simulink model "Hybrid_powertrain"  (R2021b)
settings: Solver=VariableStepAuto  StartTime=0.0  StopTime=1801  RelTol=1e-3
undefined symbols (not defined in the file): A, bvolt, C_d, discharge_mah, eff_bat, eff_dt, Eff_map, eff_map, f_rr, g, i, id, m, magnitude, Max_Torque, mu, P_aux, PM_max, r_d, rho, Ri_bat, soc_start, spd, Speed, TM_max, Torque, torque, v_reg_lim, wM_base
libraries: simulink x1, slpidlib x1
settings Model: Creator=Admin  LastModifiedBy=Admin

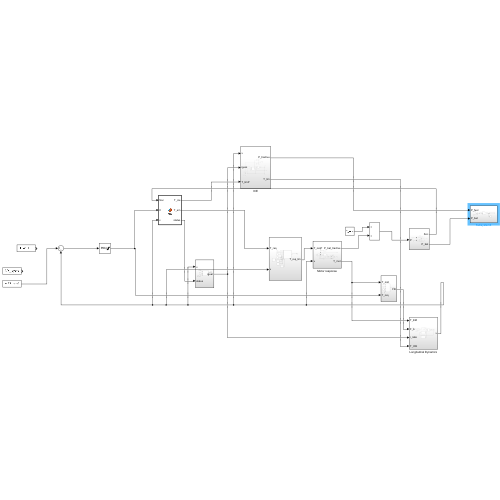
[thumbnail: Simulink's stored preview of the top-level diagram]
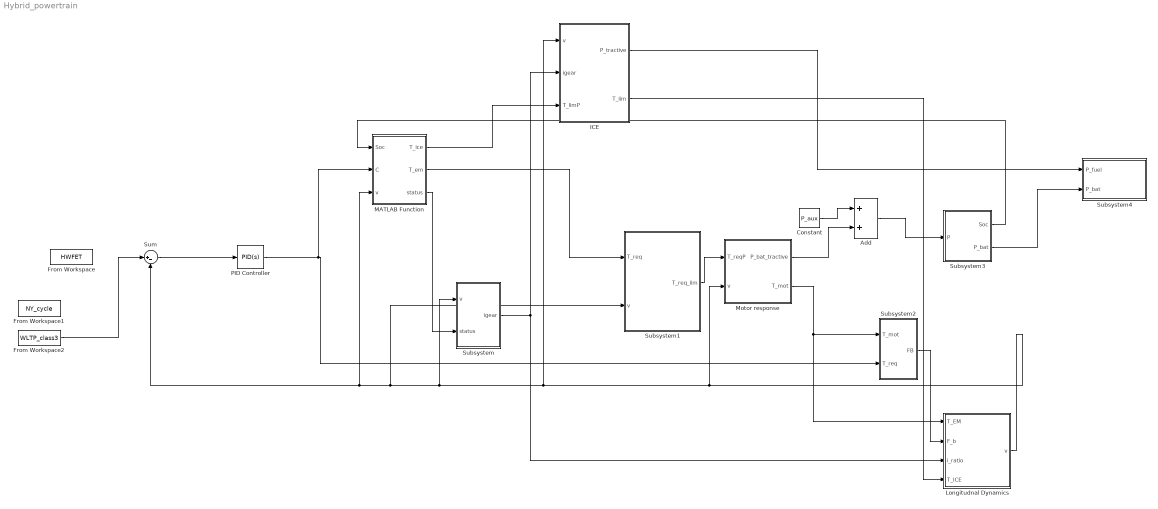
== system Hybrid_powertrain ==
  Add : Sum
  Constant : Constant  Value=P_aux
  From Workspace : FromWorkspace  VariableName=HWFET
  From Workspace1 : FromWorkspace  VariableName=NY_cycle
  From Workspace2 : FromWorkspace  VariableName=WLTP_class3
  ICE : Subsystem
  Longitudnal Dynamics : Subsystem
  MATLAB Function : MATLAB Function  TreatAsAtomicUnit=on
  Motor response : Subsystem
  PID Controller : slpidlib/PID Controller  Controller=PID  Form=Parallel  TimeDomain=Continuous-time  UseExternalTs=off  SampleTime=-1  IntegratorMethod=Forward Euler  FilterMethod=Forward Euler  ControllerParametersSource=internal  P=300  I=0  D=0  UseFilter=on  N=100  TunerSelectOption=Transfer Function Based (PID Tuner App)  InitialConditionSource=internal  InitialConditionForIntegrator=0  InitialConditionForFilter=0  DifferentiatorICPrevScaledInput=0  ExternalReset=none  TrackingMode=off  Kt=1  LimitOutput=on  SatLimitsSource=internal  UpperSaturationLimit=inf  LowerSaturationLimit=-(m*g*mu*r_d)/i  LinearizeAsGain=on  AntiWindupMode=none  Kb=1  POutMin=[]  POutMax=[]  IOutMin=[]  IOutMax=[]  DOutMin=[]  DOutMax=[]  NOutMin=[]  NOutMax=[]  SumOutMin=[]  SumOutMax=[]  SaturationOutMin=[]  SaturationOutMax=[]  PParamMin=[]  PParamMax=[]  IParamMin=[]  IParamMax=[]  DParamMin=[]  DParamMax=[]  NParamMin=[]  NParamMax=[]  KbParamMin=[]  KbParamMax=[]  KtParamMin=[]  KtParamMax=[]  KbOutMin=[]  KbOutMax=[]  KtOutMin=[]  KtOutMax=[]  IntegratorOutMin=[]  IntegratorOutMax=[]  FilterOutMin=[]  FilterOutMax=[]  SumI1OutMin=[]  SumI1OutMax=[]  SumI2OutMin=[]  SumI2OutMax=[]  SumI3OutMin=[]  SumI3OutMax=[]  SumI4OutMin=[]  SumI4OutMax=[]  SumDOutMin=[]  SumDOutMax=[]  DifferentiatorOutMin=[]  DifferentiatorOutMax=[]  FilterDiffOutCoefMin=[]  FilterDiffOutCoefMax=[]  ReciprocalOutMin=[]  ReciprocalOutMax=[]  SumDenOutMin=[]  SumDenOutMax=[]  SumNumOutMin=[]  SumNumOutMax=[]  DivideOutMin=[]  DivideOutMax=[]  UdiffTsProdOutMin=[]  UdiffTsProdOutMax=[]  NTsProdOutMin=[]  NTsProdOutMax=[]  UintegralTsProdOutMin=[]  UintegralTsProdOutMax=[]  UngainTsProdOutMin=[]  UngainTsProdOutMax=[]  IntegratorContinuousStateAttributes=''  IntegratorStateMustResolveToSignalObject=off  IntegratorRTWStateStorageClass=Auto  FilterContinuousStateAttributes=''  FilterStateMustResolveToSignalObject=off  FilterRTWStateStorageClass=Auto  ParallelPVariant=InternalParameters  IdealPVariant=Disabled  IVariant=InternalParameters  DVariant=InternalParameters  IntegratorVariant=Continuous  SatVariant=Enabled  AWVariant=Passthrough  PCopyVariant=Disabled  TRVariant=Disabled  FdbkBlocksVariant=Forward  IdealPFdbkVariant=Disabled  SatFdbkVariant=Disabled  DerivativeFilterVariant=ContFilter  NVariant=InternalParameters  NCopyVariant=Disabled  FilterICVariant=InternalICsFilter  IntegratorICVariant=InternalICs  ExternalResetVariant=Disabled  TRSumVariant=Passthrough  SumFdbkVariant=Disabled  SumVariant=Sum_PID  TsampFilterVariant=InternalTs  TsampNgainVariant=Passthrough  TsampIntegralVariant=Passthrough  ExternalSaturationOutDataTypeStr=Inherit: Same as second input
  Subsystem : Subsystem
  Subsystem1 : Subsystem
  Subsystem2 : Subsystem
  Subsystem3 : Subsystem
  Subsystem4 : Subsystem
  Sum : Sum  Inputs=|+-
  wires:
  Motor response/2(T_mot) -> Subsystem2/1(T_mot), Longitudnal Dynamics/1(T_EM)
  Sum/1 -> PID Controller/1
  Subsystem1/1(T_req_lim) -> Motor response/1(T_reqP)
  Subsystem3/2(P_bat) -> Subsystem4/2(P_bat)
  Add/1 -> Subsystem3/1(P)
  Longitudnal Dynamics/1(v) -> Motor response/2(v), ICE/1(v), Subsystem/1(v), Subsystem1/2(v), MATLAB Function/3(v), Sum/2
  Subsystem2/1(FB) -> Longitudnal Dynamics/2(F_b)
  Constant/1 -> Add/1
  Motor response/1(P_bat_tractive) -> Add/2
  PID Controller/1 -> MATLAB Function/2(C), Subsystem2/2(T_req)
  MATLAB Function/2(T_em) -> Subsystem1/1(T_req)
  MATLAB Function/3(status) -> Subsystem/2(status)
  Subsystem3/1(Soc) -> MATLAB Function/1(Soc)
  MATLAB Function/1(T_ice) -> ICE/3(T_limP)
  Subsystem/1(igear) -> Longitudnal Dynamics/3(i_ratio), ICE/2(igear)
  ICE/1(P_tractive) -> Subsystem4/1(P_fuel)
  ICE/2(T_lim) -> Longitudnal Dynamics/4(T_ICE)
  From Workspace2/1 -> Sum/1

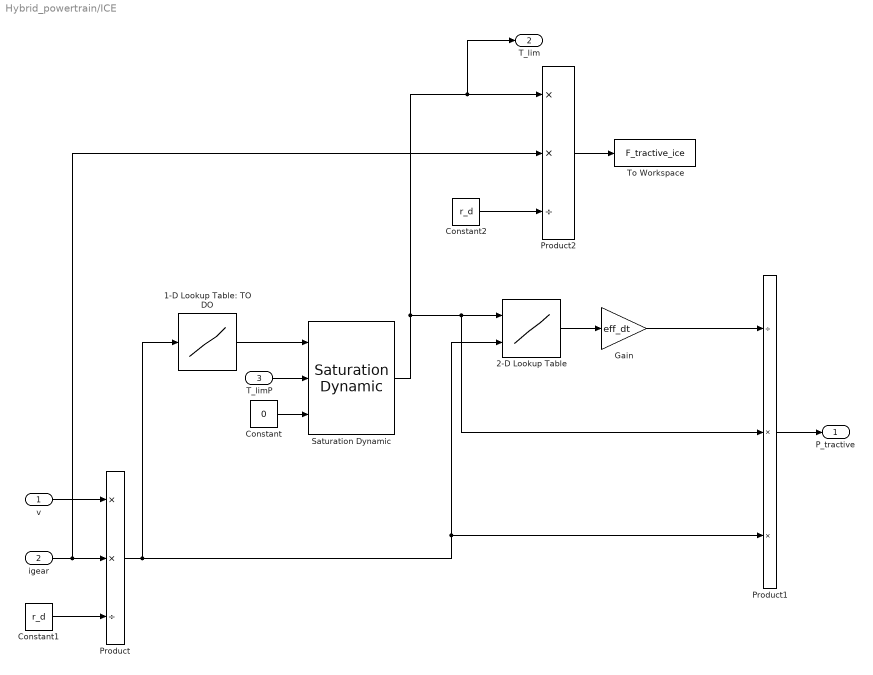
== system Hybrid_powertrain/ICE ==
  v : Inport
  igear : Inport  Port=2
  T_limP : Inport  Port=3
  "1-D Lookup Table: TO DO " : Lookup_n-D  NumberOfTableDimensions=1  BreakpointsForDimension1=Speed  Table=Max_Torque  InternalRulePriority=Speed  RndMeth=Simplest  InputSameDT=on
  2-D Lookup Table : Lookup_n-D  BreakpointsForDimension1=Torque  BreakpointsForDimension2=Speed  Table=Eff_map  InternalRulePriority=Speed  RndMeth=Simplest  InputSameDT=on
      settings: InputPortMap=u0,u1
  Constant : Constant  Value=0
  Constant1 : Constant  Value=r_d
  Constant2 : Constant  Value=r_d
  Gain : Gain  Gain=eff_dt
  Product : Product  Inputs=**/
  Product1 : Product  Inputs=/**
  Product2 : Product  Inputs=**/
  Saturation Dynamic : simulink/Discontinuities/Saturation Dynamic  OutMin=[]  OutMax=[]  OutDataTypeStr=Inherit: Same as second input  OutDataType=fixdt(1, 16)  OutScaling=2^-10  DoSatur=off
  To Workspace : ToWorkspace  VariableName=F_tractive_ice  SaveFormat=Timeseries  SampleTime=-1
  P_tractive : Outport
  T_lim : Outport  Port=2
  wires:
  v/1 -> Product/1
  igear/1 -> Product2/2, Product/2
  Constant1/1 -> Product/3
  Product/1 -> "1-D Lookup Table: TO DO "/1, 2-D Lookup Table/2, Product1/3
  Gain/1 -> Product1/1
  Constant/1 -> Saturation Dynamic/3
  T_limP/1 -> Saturation Dynamic/2
  "1-D Lookup Table: TO DO "/1 -> Saturation Dynamic/1
  2-D Lookup Table/1 -> Gain/1
  Constant2/1 -> Product2/3
  Saturation Dynamic/1 -> Product1/2, 2-D Lookup Table/1, T_lim/1, Product2/1
  Product2/1 -> To Workspace/1
  Product1/1 -> P_tractive/1

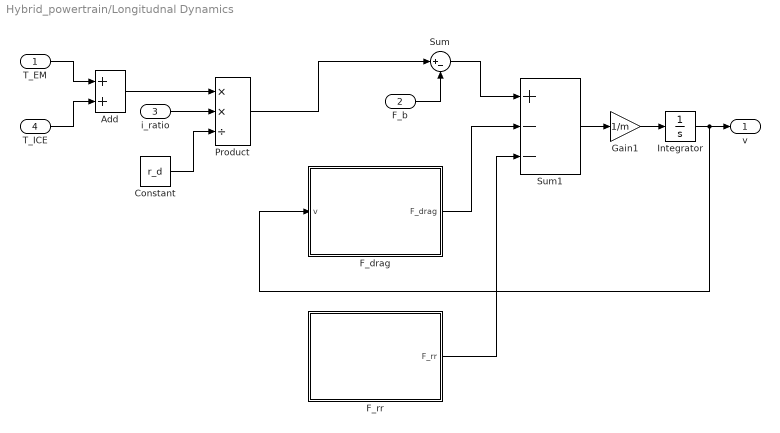
== system Hybrid_powertrain/Longitudnal Dynamics ==
  T_EM : Inport
  F_b : Inport  Port=2
  i_ratio : Inport  Port=3
  T_ICE : Inport  Port=4
  Add : Sum
  Constant : Constant  Value=r_d
  F_drag : Subsystem
  F_rr : Subsystem
  Gain1 : Gain  Gain=1/m
  Integrator : Integrator
  Product : Product  Inputs=**/
  Sum : Sum  Inputs=|+-
  Sum1 : Sum  Inputs=+--
  v : Outport
  wires:
  F_rr/1(F_rr) -> Sum1/3
  Sum1/1 -> Gain1/1
  F_b/1 -> Sum/2
  Sum/1 -> Sum1/1
  Integrator/1 -> F_drag/1(v), v/1
  Gain1/1 -> Integrator/1
  F_drag/1(F_drag) -> Sum1/2
  T_EM/1 -> Add/1
  T_ICE/1 -> Add/2
  Add/1 -> Product/1
  i_ratio/1 -> Product/2
  Constant/1 -> Product/3
  Product/1 -> Sum/1

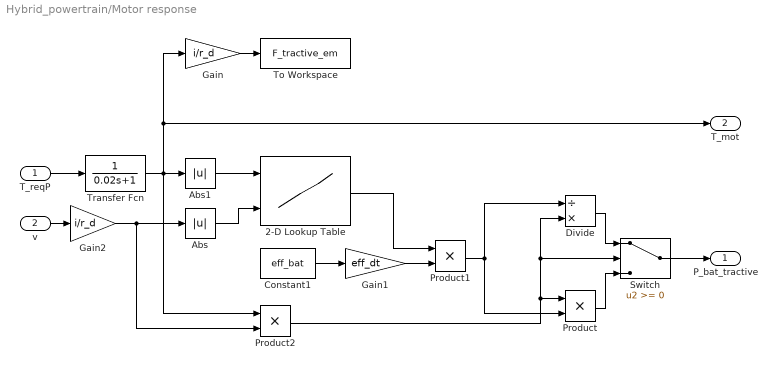
== system Hybrid_powertrain/Motor response ==
  T_reqP : Inport
  v : Inport  Port=2
  2-D Lookup Table : Lookup_n-D  BreakpointsForDimension1=torque  BreakpointsForDimension2=spd  Table=eff_map  InternalRulePriority=Speed  RndMeth=Simplest  InputSameDT=on
      settings: InputPortMap=u0,u1
  Abs : Abs
  Abs1 : Abs
  Constant1 : Constant  Value=eff_bat
  Divide : Product  Inputs=/*
  Gain : Gain  Gain=i/r_d
  Gain1 : Gain  Gain=eff_dt
  Gain2 : Gain  Gain=i/r_d
  Product : Product
  Product1 : Product
  Product2 : Product
  Switch : Switch
  To Workspace : ToWorkspace  VariableName=F_tractive_em  SaveFormat=Timeseries  SampleTime=-1
  Transfer Fcn : TransferFcn  Denominator=[0.02 1]
  P_bat_tractive : Outport
  T_mot : Outport  Port=2
  wires:
  Product/1 -> Switch/3
  v/1 -> Gain2/1
  2-D Lookup Table/1 -> Product1/1
  Divide/1 -> Switch/1
  Product1/1 -> Product/2, Divide/1
  Gain1/1 -> Product1/2
  Constant1/1 -> Gain1/1
  Abs/1 -> 2-D Lookup Table/2
  Abs1/1 -> 2-D Lookup Table/1
  Switch/1 -> P_bat_tractive/1
  Product2/1 -> Divide/2, Switch/2, Product/1
  Transfer Fcn/1 -> Gain/1, T_mot/1, Product2/1, Abs1/1
  T_reqP/1 -> Transfer Fcn/1
  Gain/1 -> To Workspace/1
  Gain2/1 -> Product2/2, Abs/1

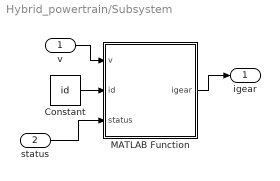
== system Hybrid_powertrain/Subsystem ==
  v : Inport
  status : Inport  Port=2
  Constant : Constant  Value=id
  MATLAB Function : MATLAB Function  TreatAsAtomicUnit=on
  igear : Outport
  wires:
  MATLAB Function/1(igear) -> igear/1
  v/1 -> MATLAB Function/1(v)
  Constant/1 -> MATLAB Function/2(id)
  status/1 -> MATLAB Function/3(status)

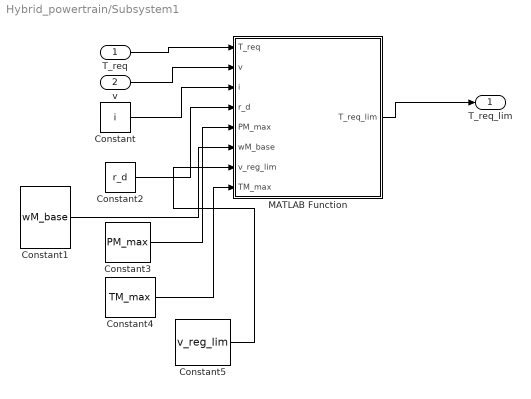
== system Hybrid_powertrain/Subsystem1 ==
  T_req : Inport
  v : Inport  Port=2
  Constant : Constant  Value=i
  Constant1 : Constant  Value=wM_base
  Constant2 : Constant  Value=r_d
  Constant3 : Constant  Value=PM_max
  Constant4 : Constant  Value=TM_max
  Constant5 : Constant  Value=v_reg_lim
  MATLAB Function : MATLAB Function  TreatAsAtomicUnit=on
  T_req_lim : Outport
  wires:
  MATLAB Function/1(T_req_lim) -> T_req_lim/1
  Constant3/1 -> MATLAB Function/5(PM_max)
  Constant/1 -> MATLAB Function/3(i)
  Constant2/1 -> MATLAB Function/4(r_d)
  v/1 -> MATLAB Function/2(v)
  T_req/1 -> MATLAB Function/1(T_req)
  Constant1/1 -> MATLAB Function/6(wM_base)
  Constant4/1 -> MATLAB Function/8(TM_max)
  Constant5/1 -> MATLAB Function/7(v_reg_lim)

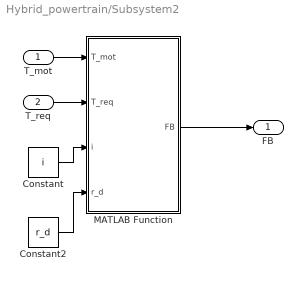
== system Hybrid_powertrain/Subsystem2 ==
  T_mot : Inport
  T_req : Inport  Port=2
  Constant : Constant  Value=i
  Constant2 : Constant  Value=r_d
  MATLAB Function : MATLAB Function  TreatAsAtomicUnit=on
  FB : Outport
  wires:
  MATLAB Function/1(FB) -> FB/1
  Constant/1 -> MATLAB Function/3(i)
  Constant2/1 -> MATLAB Function/4(r_d)
  T_req/1 -> MATLAB Function/2(T_req)
  T_mot/1 -> MATLAB Function/1(T_mot)

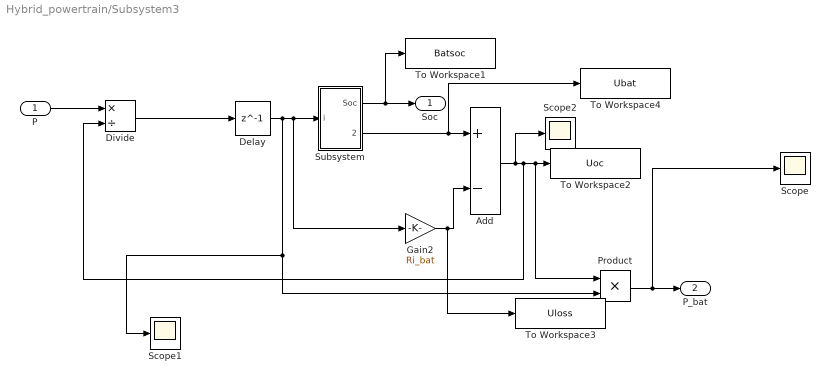
== system Hybrid_powertrain/Subsystem3 ==
  P : Inport
  Add : Sum  Inputs=+-
  Delay : Delay  DelayLength=1
  Divide : Product  Inputs=*/
  Gain2 : Gain  Gain=Ri_bat
  Product : Product
  Scope : Scope
  Scope1 : Scope
  Scope2 : Scope
  Subsystem : Subsystem
  To Workspace1 : ToWorkspace  VariableName=Batsoc  SaveFormat=Timeseries  SampleTime=-1
  To Workspace2 : ToWorkspace  VariableName=Uoc  SaveFormat=Timeseries  SampleTime=-1
  To Workspace3 : ToWorkspace  VariableName=Uloss  SaveFormat=Timeseries  SampleTime=-1
  To Workspace4 : ToWorkspace  VariableName=Ubat  SaveFormat=Timeseries  SampleTime=-1
  Soc : Outport
  P_bat : Outport  Port=2
  wires:
  Subsystem/2(Ubat) -> To Workspace4/1, Add/1
  P/1 -> Divide/1
  Delay/1 -> Scope1/1, Product/2, Gain2/1, Subsystem/1(i)
  Divide/1 -> Delay/1
  Subsystem/1(Soc) -> Soc/1, To Workspace1/1
  Add/1 -> Scope2/1, Divide/2, Product/1, To Workspace2/1
  Product/1 -> Scope/1, P_bat/1
  Gain2/1 -> To Workspace3/1, Add/2

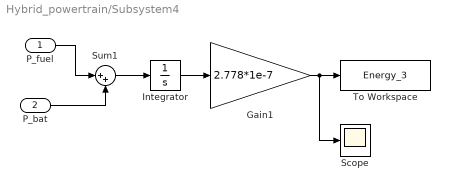
== system Hybrid_powertrain/Subsystem4 ==
  P_fuel : Inport
  P_bat : Inport  Port=2
  Gain1 : Gain  Gain=2.778*1e-7
  Integrator : Integrator
  Scope : Scope
  Sum1 : Sum  Inputs=|++
  To Workspace : ToWorkspace  VariableName=Energy_3  SaveFormat=Timeseries  SampleTime=-1
  wires:
  Integrator/1 -> Gain1/1
  Gain1/1 -> To Workspace/1, Scope/1
  P_fuel/1 -> Sum1/1
  Sum1/1 -> Integrator/1
  P_bat/1 -> Sum1/2

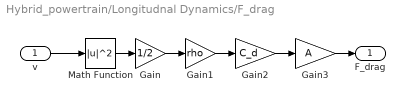
== system Hybrid_powertrain/Longitudnal Dynamics/F_drag ==
  v : Inport
  Gain : Gain  Gain=1/2
  Gain1 : Gain  Gain=rho
  Gain2 : Gain  Gain=C_d
  Gain3 : Gain  Gain=A
  Math Function : Math  Operator=magnitude^2  SaturateOnIntegerOverflow=on
  F_drag : Outport
  wires:
  Gain2/1 -> Gain3/1
  Gain/1 -> Gain1/1
  Math Function/1 -> Gain/1
  Gain1/1 -> Gain2/1
  v/1 -> Math Function/1
  Gain3/1 -> F_drag/1

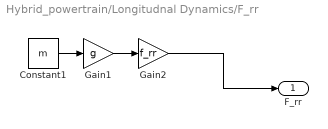
== system Hybrid_powertrain/Longitudnal Dynamics/F_rr ==
  Constant1 : Constant  Value=m
  Gain1 : Gain  Gain=g
  Gain2 : Gain  Gain=f_rr
  F_rr : Outport
  wires:
  Constant1/1 -> Gain1/1
  Gain1/1 -> Gain2/1
  Gain2/1 -> F_rr/1

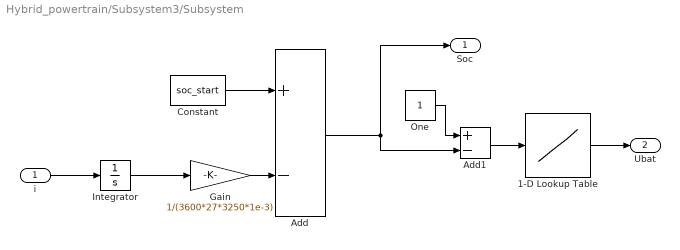
== system Hybrid_powertrain/Subsystem3/Subsystem ==
  i : Inport
  1-D Lookup Table : Lookup_n-D  NumberOfTableDimensions=1  BreakpointsForDimension1=discharge_mah  Table=bvolt  InternalRulePriority=Speed  RndMeth=Simplest  InputSameDT=on
  Add : Sum  Inputs=+-
  Add1 : Sum  Inputs=+-
  Constant : Constant  Value=soc_start
  Gain : Gain  Gain=1/(3600*27*3250*1e-3)
  Integrator : Integrator
  One : Constant  OutDataTypeStr=Inherit: Inherit via back propagation
  Soc : Outport
  Ubat : Outport  Port=2
  wires:
  Integrator/1 -> Gain/1
  Add1/1 -> 1-D Lookup Table/1
  Add/1 -> Soc/1, Add1/2
  One/1 -> Add1/1
  Gain/1 -> Add/2
  i/1 -> Integrator/1
  Constant/1 -> Add/1
  1-D Lookup Table/1 -> Ubat/1

== matlab function Hybrid_powertrain/MATLAB Function ==
  data: Soc input; T_ice output; T_em output; C input; v input; status output
function [T_ice,T_em,status] = fcn(Soc,C,v)
v = v*3.6;
if Soc > 0.5 && v < 60
    T_em = C;
    T_ice = 0;
    status = 0;
else
    if C > 0
        T_ice = C;
        T_em = 0;
        status = 1;
    else
        T_ice = 0;
        T_em = C;
        status = 0;
    end
end
end

== matlab function Hybrid_powertrain/Subsystem1/MATLAB Function ==
  data: T_req input; T_req_lim output; v input; i input; r_d input; PM_max input; wM_base input; v_reg_lim input; TM_max input
function T_req_lim = fcn(T_req,v,i,r_d,PM_max,wM_base,v_reg_lim,TM_max)

wM = (v*i)/r_d; %% angular velocity of motor
T_req_lim = T_req;

if abs(wM) > wM_base
    T_max = PM_max/wM_base;
    if abs(T_req) > T_max
        T_req_lim = sign(T_req)*T_max;
    end
elseif abs(T_req) > TM_max
   T_req_lim = sign(T_req)*TM_max;
end

if v<= v_reg_lim/3.6 & T_req_lim < 0
    T_req_lim = 0;
end

== matlab function Hybrid_powertrain/Subsystem2/MATLAB Function ==
  data: T_mot input; FB output; T_req input; i input; r_d input
function FB = fcn(T_mot,T_req,i,r_d)

if T_req<0 & T_mot>T_req
    FB = (T_mot-T_req)*(i/r_d);
else 
    FB = 0;
end
end

== matlab function Hybrid_powertrain/Subsystem/MATLAB Function ==
  data: v input; igear output; id input; status input
function igear = fcn(v,id,status)

v1 = v*3.6;
if status == 0
    igear = 9;
else
 if v1<=10
    igear = 3.07*id;
 elseif (v1>10) & (v1<=30)
    igear = 1.77*id;
 elseif (v1>30) & (v1<=50)
    igear = 1.19*id;
 elseif (v1>50) & (v1<75)
    igear = 0.87*id;
 else 
    igear = 0.7*id;
 end
end
end
